simulink model "Examen2020"  (R2022b)
settings: Solver=VariableStepAuto  StartTime=0.0  StopTime=150  MaxStep=0.01  RelTol=1e-3
libraries: slpidlib x1
settings Model: Creator=Pablo  LastModifiedBy=Pablo

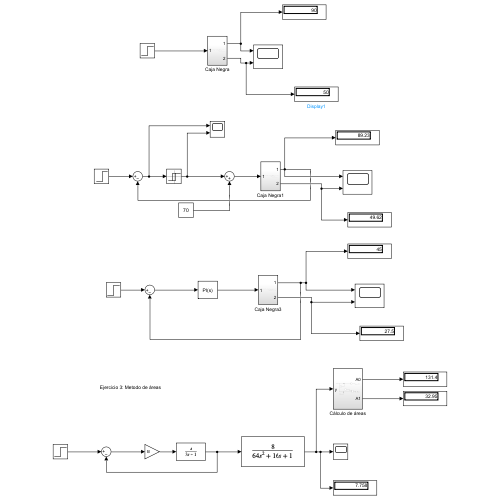
[thumbnail: Simulink's stored preview of the top-level diagram]
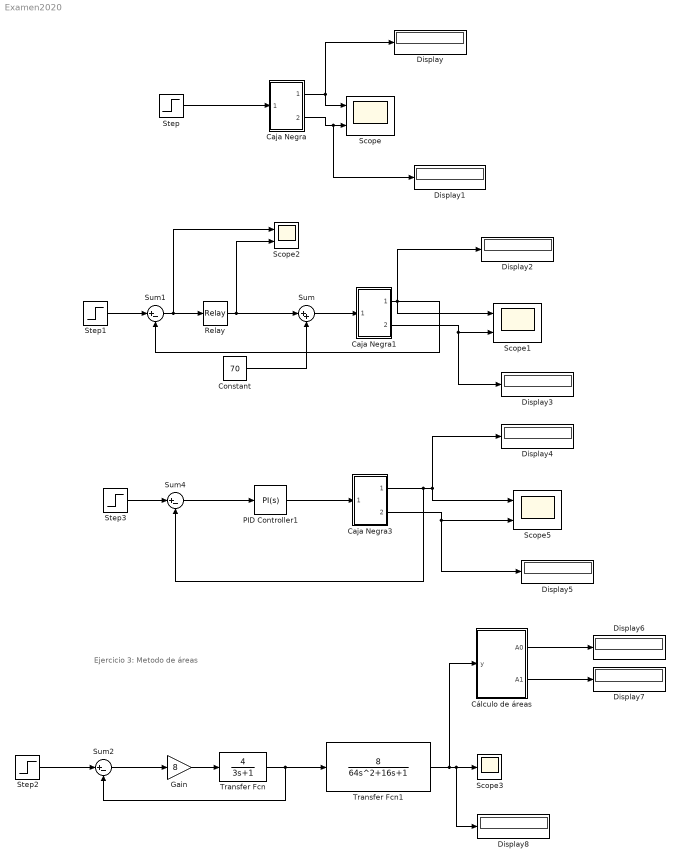
== system Examen2020 ==
  note: Ejercicio 3: Metodo de áreas
  Caja Negra : Subsystem
  Caja Negra1 : Subsystem
  Caja Negra3 : Subsystem
  Constant : Constant  Value=70
  Cálculo de áreas : Subsystem
  Display{,1..8} (9 alike) : Display
  Gain : Gain  Gain=8
  PID Controller1 : slpidlib/PID Controller  Controller=PI  Form=Ideal  TimeDomain=Continuous-time  UseExternalTs=off  SampleTime=-1  IntegratorMethod=Forward Euler  FilterMethod=Forward Euler  ControllerParametersSource=internal  P=3.296  I=1/7.152  UseKiTs=off  D=0  N=100  UseFilter=on  TunerSelectOption=Transfer Function Based (PID Tuner App)  InitialConditionSource=internal  InitialConditionForIntegrator=0  InitialConditionForFilter=0  DifferentiatorICPrevScaledInput=0  ExternalReset=none  TrackingMode=off  Kt=1  LimitOutput=off  SatLimitsSource=internal  UpperSaturationLimit=inf  LowerSaturationLimit=-inf  LinearizeAsGain=on  AntiWindupMode=none  Kb=1  LimitIntegrator=off  UpperIntegratorSaturationLimit=inf  LowerIntegratorSaturationLimit=-inf  POutMin=[]  POutMax=[]  IOutMin=[]  IOutMax=[]  DOutMin=[]  DOutMax=[]  NOutMin=[]  NOutMax=[]  SumOutMin=[]  SumOutMax=[]  SaturationOutMin=[]  SaturationOutMax=[]  PParamMin=[]  PParamMax=[]  IParamMin=[]  IParamMax=[]  DParamMin=[]  DParamMax=[]  NParamMin=[]  NParamMax=[]  KbParamMin=[]  KbParamMax=[]  KtParamMin=[]  KtParamMax=[]  KbOutMin=[]  KbOutMax=[]  KtOutMin=[]  KtOutMax=[]  IntegratorOutMin=[]  IntegratorOutMax=[]  FilterOutMin=[]  FilterOutMax=[]  SumI1OutMin=[]  SumI1OutMax=[]  SumI2OutMin=[]  SumI2OutMax=[]  SumI3OutMin=[]  SumI3OutMax=[]  SumI4OutMin=[]  SumI4OutMax=[]  SumDOutMin=[]  SumDOutMax=[]  DifferentiatorOutMin=[]  DifferentiatorOutMax=[]  FilterDiffOutCoefMin=[]  FilterDiffOutCoefMax=[]  ReciprocalOutMin=[]  ReciprocalOutMax=[]  SumDenOutMin=[]  SumDenOutMax=[]  SumNumOutMin=[]  SumNumOutMax=[]  DivideOutMin=[]  DivideOutMax=[]  UdiffTsProdOutMin=[]  UdiffTsProdOutMax=[]  NTsProdOutMin=[]  NTsProdOutMax=[]  UintegralTsProdOutMin=[]  UintegralTsProdOutMax=[]  UngainTsProdOutMin=[]  UngainTsProdOutMax=[]  ClampingZeroOutDataTypeStr=Inherit: Inherit via back propagation  ClampingZeroOutMin=[]  ClampingZeroOutMax=[]  FilterDenConstantOutDataTypeStr=Inherit: Inherit via back propagation  FilterDenConstantOutMin=[]  FilterDenConstantOutMax=[]  PCopyOutDataTypeStr=Inherit: Inherit via back propagation  PCopyOutMin=[]  PCopyOutMax=[]  NCopyOutDataTypeStr=Inherit: Inherit via back propagation  NCopyOutMin=[]  NCopyOutMax=[]  IntegratorContinuousStateAttributes=''  IntegratorStateMustResolveToSignalObject=off  IntegratorRTWStateStorageClass=Auto  FilterContinuousStateAttributes=''  FilterStateMustResolveToSignalObject=off  FilterRTWStateStorageClass=Auto  ParallelPVariant=Passthrough  IdealPVariant=InternalParameters  IVariant=InternalParameters  DVariant=Disabled  IntegratorVariant=Continuous  SatVariant=Disabled  AWVariant=Passthrough  PCopyVariant=Disabled  TRVariant=Disabled  FdbkBlocksVariant=Forward  IdealPFdbkVariant=Disabled  SatFdbkVariant=Disabled  DerivativeFilterVariant=Disabled  NVariant=Disabled  NCopyVariant=Disabled_SignalSpec  FilterICVariant=Disabled  IntegratorICVariant=InternalICs  ExternalResetVariant=Disabled  TRSumVariant=Passthrough  SumFdbkVariant=Disabled  SumVariant=Sum_PI  TsampFilterVariant=InternalTs  TsampNgainVariant=Passthrough  TsampIntegralVariant=Passthrough  ExternalSaturationOutDataTypeStr=Inherit: Same as second input
  Relay : Relay  OnOutputValue=5  OffOutputValue=-5
  Scope{,1..2,5} (4 alike) : Scope  NumInputPorts=2
  Scope3 : Scope
  Step : Step  After=70  SampleTime=0
  Step1 : Step  After=90  SampleTime=0
  Step2 : Step  SampleTime=0
  Step3 : Step  After=45  SampleTime=0
  Sum : Sum  Inputs=|++
  Sum1 : Sum  Inputs=|+-
  Sum2 : Sum  Inputs=|+-
  Sum4 : Sum  Inputs=|+-
  Transfer Fcn : TransferFcn  Numerator=[4]  Denominator=[3 1]
  Transfer Fcn1 : TransferFcn  Numerator=[8]  Denominator=[64 16 1]
  wires:
  Caja Negra/1(Out1) -> Display/1, Scope/1
  Step/1 -> Caja Negra/1(In1)
  Caja Negra/2(Output) -> Display1/1, Scope/2
  Caja Negra1/2(Output) -> Scope1/2, Display3/1
  Caja Negra1/1(Out1) -> Scope1/1, Display2/1, Sum1/2
  Relay/1 -> Scope2/2, Sum/1
  Sum/1 -> Caja Negra1/1(In1)
  Constant/1 -> Sum/2
  Sum1/1 -> Scope2/1, Relay/1
  Step1/1 -> Sum1/1
  Step3/1 -> Sum4/1
  Caja Negra3/2(Output) -> Scope5/2, Display5/1
  Caja Negra3/1(Out1) -> Sum4/2, Scope5/1, Display4/1
  Sum4/1 -> PID Controller1/1
  PID Controller1/1 -> Caja Negra3/1(In1)
  Gain/1 -> Transfer Fcn/1
  Sum2/1 -> Gain/1
  Transfer Fcn/1 -> Transfer Fcn1/1, Sum2/2
  Step2/1 -> Sum2/1
  Transfer Fcn1/1 -> Cálculo de áreas/1(y), Display8/1, Scope3/1
  Cálculo de áreas/1(A0) -> Display6/1
  Cálculo de áreas/2(A1) -> Display7/1

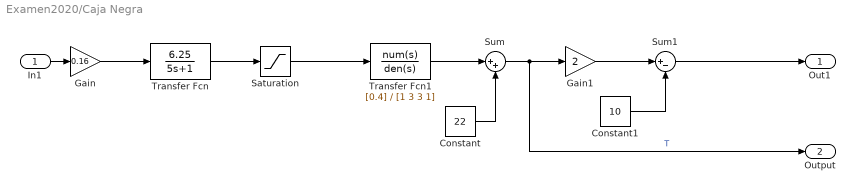
== system Examen2020/Caja Negra ==
  In1 : Inport
  Constant : Constant  Value=22
  Constant1 : Constant  Value=10
  Gain : Gain  Gain=0.16
  Gain1 : Gain  Gain=2
  Saturation : Saturate  UpperLimit=100  LowerLimit=0
  Sum : Sum  Inputs=|++
  Sum1 : Sum  Inputs=|+-
  Transfer Fcn : TransferFcn  Numerator=[6.25]  Denominator=[5 1]
  Transfer Fcn1 : TransferFcn  Numerator=[0.4]  Denominator=[1 3 3 1]
  Out1 : Outport
  Output : Outport  Port=2
  wires:
  Constant/1 -> Sum/2
  Gain/1 -> Transfer Fcn/1
  Gain1/1 -> Sum1/1
  Sum/1 -> Output/1, Gain1/1  "T"
  Transfer Fcn1/1 -> Sum/1
  Constant1/1 -> Sum1/2
  Saturation/1 -> Transfer Fcn1/1
  Transfer Fcn/1 -> Saturation/1
  Sum1/1 -> Out1/1
  In1/1 -> Gain/1

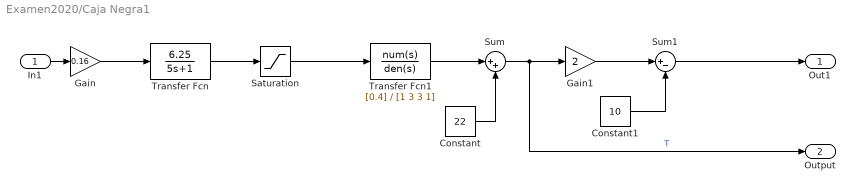
== system Examen2020/Caja Negra1 ==
  In1 : Inport
  Constant : Constant  Value=22
  Constant1 : Constant  Value=10
  Gain : Gain  Gain=0.16
  Gain1 : Gain  Gain=2
  Saturation : Saturate  UpperLimit=100  LowerLimit=0
  Sum : Sum  Inputs=|++
  Sum1 : Sum  Inputs=|+-
  Transfer Fcn : TransferFcn  Numerator=[6.25]  Denominator=[5 1]
  Transfer Fcn1 : TransferFcn  Numerator=[0.4]  Denominator=[1 3 3 1]
  Out1 : Outport
  Output : Outport  Port=2
  wires:
  Constant/1 -> Sum/2
  Gain/1 -> Transfer Fcn/1
  Gain1/1 -> Sum1/1
  Sum/1 -> Output/1, Gain1/1  "T"
  Transfer Fcn1/1 -> Sum/1
  Constant1/1 -> Sum1/2
  Saturation/1 -> Transfer Fcn1/1
  Transfer Fcn/1 -> Saturation/1
  Sum1/1 -> Out1/1
  In1/1 -> Gain/1

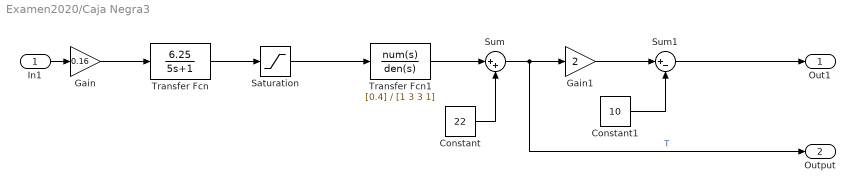
== system Examen2020/Caja Negra3 ==
  In1 : Inport
  Constant : Constant  Value=22
  Constant1 : Constant  Value=10
  Gain : Gain  Gain=0.16
  Gain1 : Gain  Gain=2
  Saturation : Saturate  UpperLimit=100  LowerLimit=0
  Sum : Sum  Inputs=|++
  Sum1 : Sum  Inputs=|+-
  Transfer Fcn : TransferFcn  Numerator=[6.25]  Denominator=[5 1]
  Transfer Fcn1 : TransferFcn  Numerator=[0.4]  Denominator=[1 3 3 1]
  Out1 : Outport
  Output : Outport  Port=2
  wires:
  Constant/1 -> Sum/2
  Gain/1 -> Transfer Fcn/1
  Gain1/1 -> Sum1/1
  Sum/1 -> Output/1, Gain1/1  "T"
  Transfer Fcn1/1 -> Sum/1
  Constant1/1 -> Sum1/2
  Saturation/1 -> Transfer Fcn1/1
  Transfer Fcn/1 -> Saturation/1
  Sum1/1 -> Out1/1
  In1/1 -> Gain/1

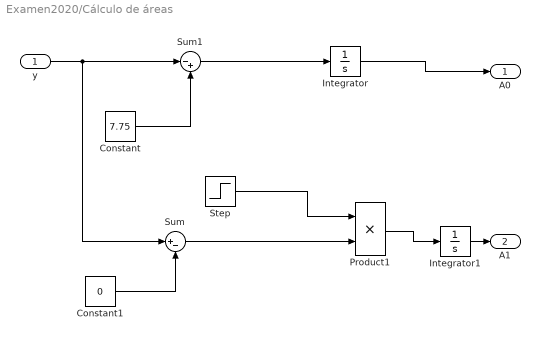
== system Examen2020/Cálculo de áreas ==
  y : Inport
  Constant : Constant  Value=7.75
  Constant1 : Constant  Value=0
  Integrator : Integrator
  Integrator1 : Integrator
  Product1 : Product
  Step : Step  Time=16.95  Before=1  After=0  SampleTime=0
  Sum : Sum  Inputs=|+-
  Sum1 : Sum  Inputs=|-+
  A0 : Outport
  A1 : Outport  Port=2
  wires:
  Step/1 -> Product1/1
  Sum/1 -> Product1/2
  Integrator1/1 -> A1/1
  Product1/1 -> Integrator1/1
  Sum1/1 -> Integrator/1
  Constant/1 -> Sum1/2
  Constant1/1 -> Sum/2
  Integrator/1 -> A0/1
  y/1 -> Sum/1, Sum1/1
